simulink model "Converter_DC_motor_drive_CLC"  (R2016b)
settings: Solver=VariableStepAuto  StartTime=0.0  StopTime=100  RelTol=1e-3
PreLoadFcn:
  | a=0;
  | b=a*0.01/180;
libraries: powerlib x11, powerlib_meascontrol x3, simulink x1
settings Model: Creator=acer  LastModifiedBy=acer

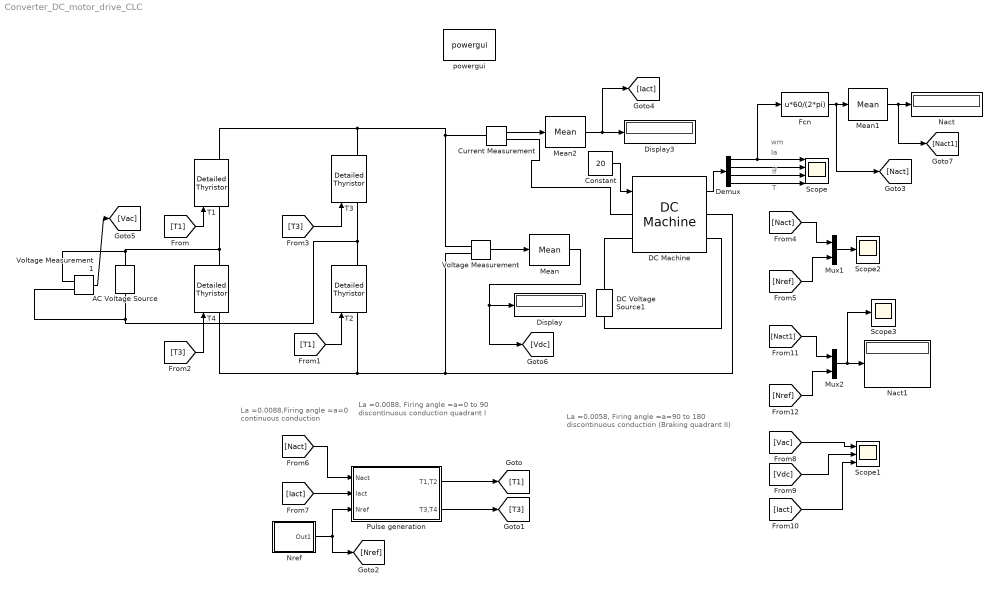
== system Converter_DC_motor_drive_CLC ==
  note: T
  note: If
  note: Ia
  note: wm
  note: La =0.0088,Firing angle =a=0
      | continuous conduction
  note: La =0.0088, Firing angle =a=0 to 90
      | discontinuous conduction quadrant I
  note: La =0.0058, Firing angle =a=90 to 180
      | discontinuous conduction (Braking quadrant II)
  AC Voltage Source : powerlib/Electrical Sources/AC Voltage Source  Amplitude=230*sqrt(2)  Phase=0  Frequency=50  SampleTime=0  Measurements=None  BusType=swing  Pref=10e3  Qref=0  Qmin=-inf  Qmax=+inf
  Constant : Constant  Value=20
  Current Measurement : powerlib/Measurements/Current Measurement  PhasorSimulation=off  OutputType=Complex  PSBequivalent=0
  DC Machine : powerlib/Machines/DC Machine  PresetModel=No  MechanicalLoad=Torque TL  FieldType=Wound  ShowDetailedParameters=on  MeasurementBus=off  RLa=[2.581 0.0058]  RLf=[281.3 156]  Laf=0.9483  MachineConstant=Torque constant (N.m/A)  Ke=1.8  Kt=1.8  J=0.02215  Bm=0.002953  Tf=0.5161  w0=0  Ifinit=0  TsPowergui=0  TsBlock=-1
  DC Voltage Source1 : powerlib/Electrical Sources/DC Voltage Source  Amplitude=240  Measurements=None
  Demux : Demux
  Display : Display
  Display3 : Display
  Fcn : Fcn  Expr=u*60/(2*pi)
  Mean : powerlib_meascontrol/Measurements/Mean  Freq=50  Vinit=0  Ts=0
  Mean1 : powerlib_meascontrol/Measurements/Mean  Freq=50  Vinit=0  Ts=0
  Mean2 : powerlib_meascontrol/Measurements/Mean  Freq=50  Vinit=0  Ts=0
  Mux1 : Mux  Inputs=2
  Mux2 : Mux  Inputs=2
  Nact : Display
  Nact1 : Display
  Nref : Subsystem
  Pulse generation : Subsystem
  Scope : Scope  NumInputPorts=4
  Scope1 : Scope  NumInputPorts=3
  Scope2 : Scope
  Scope3 : Scope
  T1 : powerlib/Power Electronics/Detailed Thyristor  Ron=0.001  Lon=1e-3  Vf=0  IL=0  Tq=1e-9  IC=0  Rs=500  Cs=250e-9  Measurements=on
  T2 : powerlib/Power Electronics/Detailed Thyristor  Ron=0.001  Lon=1e-3  Vf=0  IL=0  Tq=1e-9  IC=0  Rs=500  Cs=250e-9  Measurements=on
  T3 : powerlib/Power Electronics/Detailed Thyristor  Ron=0.001  Lon=1e-3  Vf=0  IL=0.1  Tq=1e-6  IC=0  Rs=500  Cs=250e-9  Measurements=on
  T4 : powerlib/Power Electronics/Detailed Thyristor  Ron=0.001  Lon=1e-3  Vf=0  IL=0.1  Tq=1e-6  IC=0  Rs=500  Cs=250e-9  Measurements=on
  Voltage Measurement : powerlib/Measurements/Voltage Measurement  PhasorSimulation=off  OutputType=Complex  PSBequivalent=0
  Voltage Measurement1 : powerlib/Measurements/Voltage Measurement  PhasorSimulation=off  OutputType=Complex  PSBequivalent=0
  powergui : powerlib/powergui  Priority=1  SimulationMode=Discrete  SolverType=Tustin/Backward Euler (TBE)  SampleTime=50e-6  frequency=60  SPID=off  DisableSnubberDevices=off  DisableRonSwitches=off  DisableVfSwitches=off  SwTol=0  DisplayEquations=off  Interpol=off  ExternalGateDelay=off  methode=off  Ts=10  FunctionMessages=off  echomessages=off  HookPort=off  EnableUseOfTLC=off  x0status=blocks  frequencyindice=0  Pbase=100e6  ErrMax=1e-4  Iterations=50  UnitsV=kV  UnitsW=MW  buscounter=0  RestoreLinks=warning  ResistiveCurrentMeasurement=off  Frange=[0:2:500]  Ylog=off  Xlog=on  ShowGrid=off  save=off  variable=ZData  structure=0  ZoomFFT=off  StartTime=0.0  cycles=1  DisplayStyle=1  fundamental=60  FreqAxis=off  MaxFrequency=1000  frequencyindicesteady=1  RmsSteady=1  display=off
  wires:
  Constant/1 -> DC Machine/1
  DC Machine/1 -> Demux/1
  Demux/1 -> Fcn/1, Scope/1
  Demux/3 -> Scope/3
  Demux/4 -> Scope/4
  Current Measurement/1 -> Mean2/1
  Demux/2 -> Scope/2
  Mean1/1 -> [Nact1], Nact/1
  Mean2/1 -> [Iact], Display3/1
  Nref/1(Out1) -> Pulse generation/3(Nref), [Nref]
  Fcn/1 -> [Nact], Mean1/1
  Pulse generation/1(T1,T2) -> [T1]
  Pulse generation/2(T3,T4) -> [T3]
  [T1] -> T1/1
  [T1] -> T2/1
  [T3] -> T4/1
  [T3] -> T3/1
  [Nact] -> Mux1/1
  [Nref] -> Mux1/2
  [Nact] -> Pulse generation/1(Nact)
  [Iact] -> Pulse generation/2(Iact)
  Voltage Measurement/1 -> Mean/1
  Mean/1 -> [Vdc], Display/1
  Voltage Measurement1/1 -> [Vac]
  [Vac] -> Scope1/1
  [Vdc] -> Scope1/2
  [Iact] -> Scope1/3
  Mux1/1 -> Scope2/1
  [Nact1] -> Mux2/1
  [Nref] -> Mux2/2
  Mux2/1 -> Scope3/1, Nact1/1
  connections:
  DC Voltage Source1/RConn1 -- DC Machine/LConn2
  DC Voltage Source1/LConn1 -- DC Machine/RConn2
  T4/RConn1 -- Voltage Measurement1/LConn1 -- AC Voltage Source/RConn1 -- T1/LConn1
  T2/RConn1 -- Voltage Measurement1/LConn2 -- AC Voltage Source/LConn1 -- T3/LConn1
  T3/RConn1 -- Current Measurement/LConn1 -- Voltage Measurement/LConn1 -- T1/RConn1
  T4/LConn1 -- DC Machine/RConn1 -- Voltage Measurement/LConn2 -- T2/LConn1
  Current Measurement/RConn1 -- DC Machine/LConn1

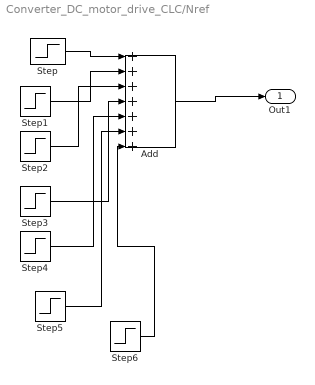
== system Converter_DC_motor_drive_CLC/Nref ==
  Add : Sum  Inputs=+++++++
  Step : Step  Time=10  Before=800  After=500  SampleTime=0
  Step1 : Step  Time=20  After=100  SampleTime=0
  Step2 : Step  Time=30  After=100  SampleTime=0
  Step3 : Step  Time=40  After=100  SampleTime=0
  Step4 : Step  Time=50  After=-350  SampleTime=0
  Step5 : Step  Time=60  After=450  SampleTime=0
  Step6 : Step  Time=70  After=100  SampleTime=0
  Out1 : Outport
  wires:
  Step/1 -> Add/1
  Step1/1 -> Add/2
  Step2/1 -> Add/3
  Step3/1 -> Add/4
  Step4/1 -> Add/5
  Step5/1 -> Add/6
  Step6/1 -> Add/7
  Add/1 -> Out1/1

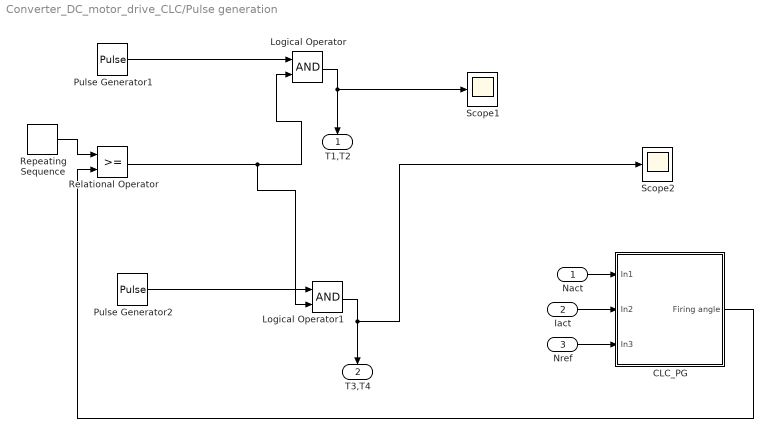
== system Converter_DC_motor_drive_CLC/Pulse generation ==
  Nact : Inport
  Iact : Inport  Port=2
  Nref : Inport  Port=3
  CLC_PG : Subsystem
  Logical Operator : Logic  AllPortsSameDT=off  OutDataTypeStr=boolean
  Logical Operator1 : Logic  AllPortsSameDT=off  OutDataTypeStr=boolean
  Pulse Generator1 : DiscretePulseGenerator  PulseType=Time based  Period=0.02  PulseWidth=50
  Pulse Generator2 : DiscretePulseGenerator  PulseType=Time based  Period=0.02  PulseWidth=50  PhaseDelay=0.01
  Relational Operator : RelationalOperator  OutDataTypeStr=boolean  RndMeth=Simplest
  Repeating Sequence : simulink/Sources/Repeating Sequence  rep_seq_t=[0 0.01]  rep_seq_y=[0 0.005]
  Scope1 : Scope
  Scope2 : Scope
  T1,T2 : Outport
  T3,T4 : Outport  Port=2
  wires:
  Pulse Generator1/1 -> Logical Operator/1
  Repeating Sequence/1 -> Relational Operator/1
  Logical Operator/1 -> T1,T2/1, Scope1/1
  Pulse Generator2/1 -> Logical Operator1/1
  Logical Operator1/1 -> Scope2/1, T3,T4/1
  Relational Operator/1 -> Logical Operator1/2, Logical Operator/2
  Nact/1 -> CLC_PG/1(In1)
  Iact/1 -> CLC_PG/2(In2)
  Nref/1 -> CLC_PG/3(In3)
  CLC_PG/1(Firing angle) -> Relational Operator/2

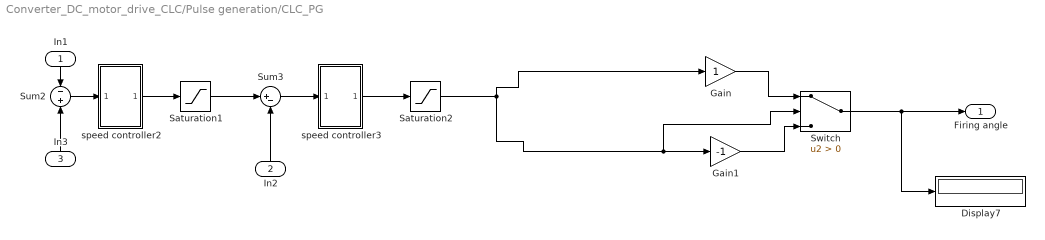
== system Converter_DC_motor_drive_CLC/Pulse generation/CLC_PG ==
  In1 : Inport
  In2 : Inport  Port=2
  In3 : Inport  Port=3
  Display7 : Display
  Gain : Gain
  Gain1 : Gain  Gain=-1
  Saturation1 : Saturate  UpperLimit=30  LowerLimit=-30
  Saturation2 : Saturate  UpperLimit=1  LowerLimit=-1
  Sum2 : Sum  Inputs=-+
  Sum3 : Sum  Inputs=|+-
  Switch : Switch  Criteria=u2 > Threshold
  speed controller2 : Subsystem
  speed controller3 : Subsystem
  Firing angle : Outport
  wires:
  Sum3/1 -> speed controller3/1(In1)
  speed controller3/1(Out1) -> Saturation2/1
  In1/1 -> Sum2/1
  Saturation1/1 -> Sum3/1
  In2/1 -> Sum3/2
  Sum2/1 -> speed controller2/1(In1)
  Saturation2/1 -> Gain/1, Switch/2, Gain1/1
  speed controller2/1(Out1) -> Saturation1/1
  Gain/1 -> Switch/1
  Gain1/1 -> Switch/3
  Switch/1 -> Display7/1, Firing angle/1
  In3/1 -> Sum2/2

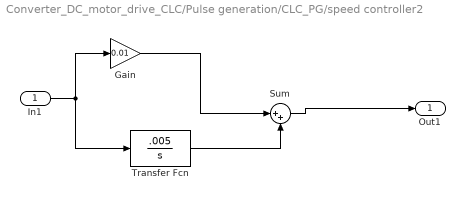
== system Converter_DC_motor_drive_CLC/Pulse generation/CLC_PG/speed controller2 ==
  In1 : Inport
  Gain : Gain  Gain=0.01
  Sum : Sum  Inputs=|++
  Transfer Fcn : TransferFcn  Numerator=[.005]  Denominator=[1 0]
  Out1 : Outport
  wires:
  In1/1 -> Gain/1, Transfer Fcn/1
  Gain/1 -> Sum/1
  Transfer Fcn/1 -> Sum/2
  Sum/1 -> Out1/1

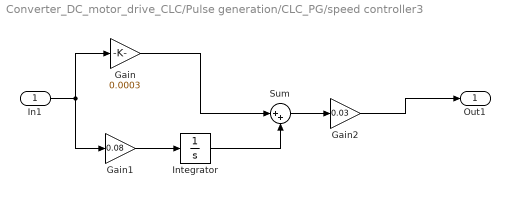
== system Converter_DC_motor_drive_CLC/Pulse generation/CLC_PG/speed controller3 ==
  In1 : Inport
  Gain : Gain  Gain=0.0003
  Gain1 : Gain  Gain=0.08
  Gain2 : Gain  Gain=0.03
  Integrator : Integrator
  Sum : Sum  Inputs=|++
  Out1 : Outport
  wires:
  Sum/1 -> Gain2/1
  In1/1 -> Gain/1, Gain1/1
  Gain1/1 -> Integrator/1
  Gain/1 -> Sum/1
  Integrator/1 -> Sum/2
  Gain2/1 -> Out1/1
